simulink model "test_pos_ctrl_target_for_each"  (R2014a)
settings: Solver=ode5  StartTime=0.0  StopTime=inf  FixedStep=basic_time_step  RelTol=1e-3
values from neighbouring files (symbols this model uses):
  basic_time_step = 0.002    [init_pos_ctrl_target_for_each.m]
  g = 9.81    [init_pos_ctrl_target_for_each.m]
  kd = [2 0 0 ... (first row only)    [init_pos_ctrl_target_for_each.m]
  KDP = 11/5    (= 2.2)    [init_pos_ctrl_target_for_each.m]
  KDR = 11/5    (= 2.2)    [init_pos_ctrl_target_for_each.m]
  KDY = 11    [init_pos_ctrl_target_for_each.m]
  ki = 0*[.1 0 0 ... (first row only)    [init_pos_ctrl_target_for_each.m]
  kp = [1 0 0 ... (first row only)    [init_pos_ctrl_target_for_each.m]
  KPP = 30/5    (= 6)    [init_pos_ctrl_target_for_each.m]
  KPR = 30/5    (= 6)    [init_pos_ctrl_target_for_each.m]
  KPY = 30    [init_pos_ctrl_target_for_each.m]
  m0 = 1.3    [init_pos_ctrl_target_for_each.m]
  max_pitch = sin(15*pi/180)    [init_pos_ctrl_target_for_each.m]
  max_roll = sin(15*pi/180)    [init_pos_ctrl_target_for_each.m]
  n_robots = 1    [init_pos_ctrl_target_for_each.m]
undefined symbols (not defined in the file or in its folder): DiscIntNeverNeededParam, IMU_time_step, VICON_time_step
libraries: geometry_msgs x3, sensor_msgs x1, rt_sync x1
settings Model: Creator=prg  LastModifiedBy=fschiano
settings OptimizationCC: ExpressionDepthLimit=2147483647
settings DebuggingCC: UnderspecifiedInitializationDetection=Classic  StateNameClashWarn=warning

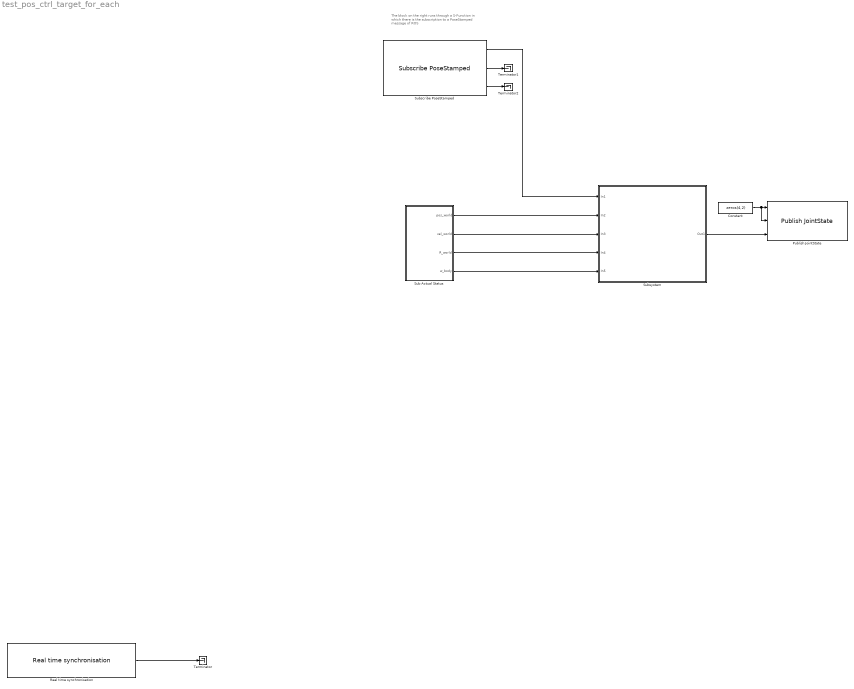
== system test_pos_ctrl_target_for_each ==
  note: The block on the right runs through a S-Function
      | in which there is the subscription to a PoseStamped
      | message of ROS
  Constant : Constant  Value=zeros(4,2)
  Publish JointState : sensor_msgs/Publish JointState  stepTime=basic_time_step  topic_prefix='/command/quadrotor_'  list_of_robot_ids=char([0:1])  topic_postfix=''  n_dofs=char(4)
  Real time synchronisation : rt_sync/Real time synchronisation  stepTime=basic_time_step  minShownDelay=0.5  ShowEveryNumCycles=1/basic_time_step  slowDownFactor=1
  Sub Actual Status : Subsystem
  Subscribe PoseStamped : geometry_msgs/Subscribe PoseStamped  stepTime=basic_time_step  topic_prefix='/vrep/Quadricopter_target_'  list_of_robot_ids=char([0:1])  topic_postfix='/pose'
  Subsystem : Subsystem
  Terminator : Terminator
  Terminator1 : Terminator
  Terminator2 : Terminator
  wires:
  Constant/1 -> Publish JointState/2, Publish JointState/1
  Real time synchronisation/1 -> Terminator/1
  Subscribe PoseStamped/2 -> Terminator1/1
  Subscribe PoseStamped/3 -> Terminator2/1
  Subscribe PoseStamped/1 -> Subsystem/1(In1)
  Sub Actual Status/1(pos_world) -> Subsystem/2(In2)
  Sub Actual Status/2(vel_world) -> Subsystem/3(In3)
  Sub Actual Status/3("R_world ") -> Subsystem/4(In4)
  Sub Actual Status/4(w_body) -> Subsystem/5(In5)
  Subsystem/1(Out1) -> Publish JointState/3

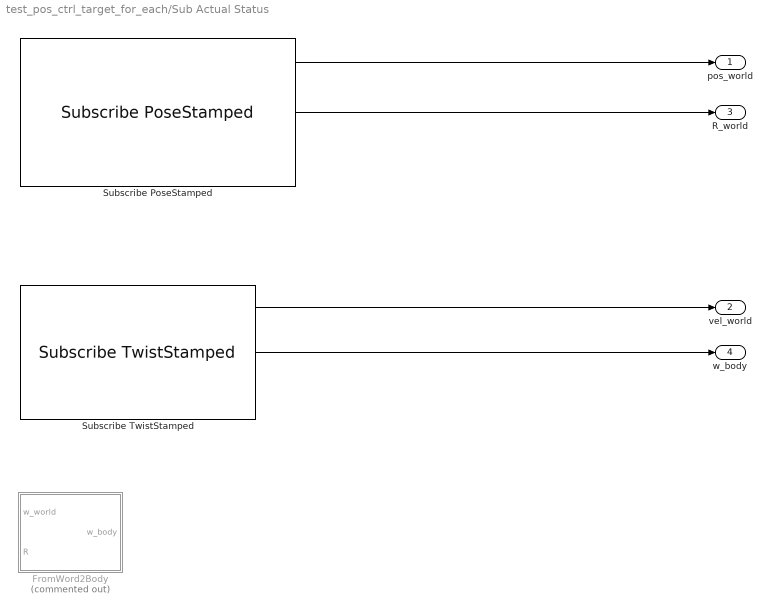
== system test_pos_ctrl_target_for_each/Sub Actual Status ==
  FromWord2Body : MATLAB Function  Commented=on  TreatAsAtomicUnit=on
  Subscribe PoseStamped : geometry_msgs/Subscribe PoseStamped  stepTime=basic_time_step  topic_prefix='/vrep/pose/quadrotor_'  list_of_robot_ids=char([0:1])  topic_postfix=''
  Subscribe TwistStamped : geometry_msgs/Subscribe TwistStamped  stepTime=basic_time_step  topic_prefix='/vrep/twist/quadrotor_'  list_of_robot_ids=char([0:1])  topic_postfix=''
  pos_world : Outport
  vel_world : Outport  Port=2
  "R_world " : Outport  Port=3
  w_body : Outport  Port=4
  wires:
  Subscribe PoseStamped/1 -> pos_world/1
  Subscribe PoseStamped/2 -> "R_world "/1
  Subscribe TwistStamped/1 -> vel_world/1
  Subscribe TwistStamped/2 -> w_body/1

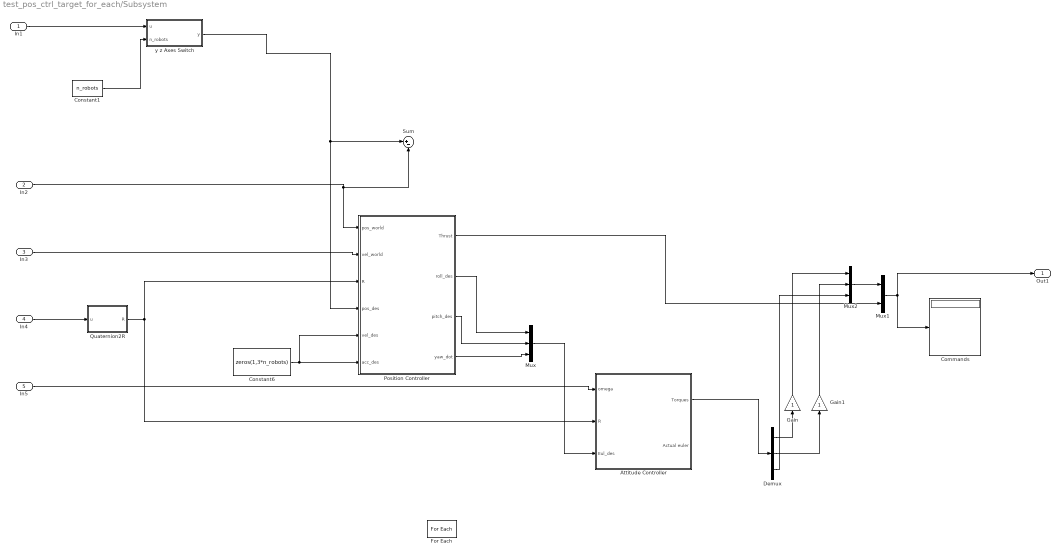
== system test_pos_ctrl_target_for_each/Subsystem ==
  In1 : Inport  Partition=on  PartitionDimension=2  PartitionWidth=1
  In2 : Inport  Port=2  Partition=on  PartitionDimension=2  PartitionWidth=1
  In3 : Inport  Port=3  Partition=on  PartitionDimension=2  PartitionWidth=1
  In4 : Inport  Port=4  Partition=on  PartitionDimension=2  PartitionWidth=1
  In5 : Inport  Port=5  Partition=on  PartitionDimension=2  PartitionWidth=1
  Attitude Controller : Subsystem  SystemSampleTime=IMU_time_step
  Commands : Display
  Constant1 : Constant  Value=n_robots
  Constant6 : Constant  Value=zeros(1,3*n_robots)
  Demux : Demux  Outputs=3
  For Each : ForEach  DisableCoverage=on  IndexMode=One-based
  Gain : Gain
  Gain1 : Gain
  Mux : Mux  Inputs=3
  Mux1 : Mux  Inputs=2
  Mux2 : Mux  Inputs=3
  Position Controller : Subsystem  SystemSampleTime=VICON_time_step
  Quaternion2R : MATLAB Function  TreatAsAtomicUnit=on
  Sum : Sum  Inputs=|+-
  y z Axes Switch : MATLAB Function  TreatAsAtomicUnit=on
  Out1 : Outport  ConcatenationDimension=2
  wires:
  Demux/2 -> Gain1/1
  Demux/3 -> Mux2/3
  Mux2/1 -> Mux1/1
  Mux1/1 -> Out1/1, Commands/1
  y z Axes Switch/1(y) -> Position Controller/4(pos_des), Sum/1
  Gain1/1 -> Mux2/2
  In3/1 -> Position Controller/2(vel_world)
  In4/1 -> Quaternion2R/1(u)
  Position Controller/1(Thrust) -> Mux1/2
  In2/1 -> Sum/2, Position Controller/1(pos_world)
  Position Controller/4(yaw_dot) -> Mux/3
  Constant6/1 -> Position Controller/5(vel_des), Position Controller/6(acc_des)
  Mux/1 -> Attitude Controller/3(Eul_des)
  Demux/1 -> Gain/1
  Position Controller/2(roll_des) -> Mux/1
  Position Controller/3(pitch_des) -> Mux/2
  Gain/1 -> Mux2/1
  Constant1/1 -> y z Axes Switch/2(n_robots)
  Attitude Controller/1(Torques) -> Demux/1
  In5/1 -> Attitude Controller/1(omega)
  In1/1 -> y z Axes Switch/1(u)
  Quaternion2R/1(R) -> Attitude Controller/2(R), Position Controller/3(R)

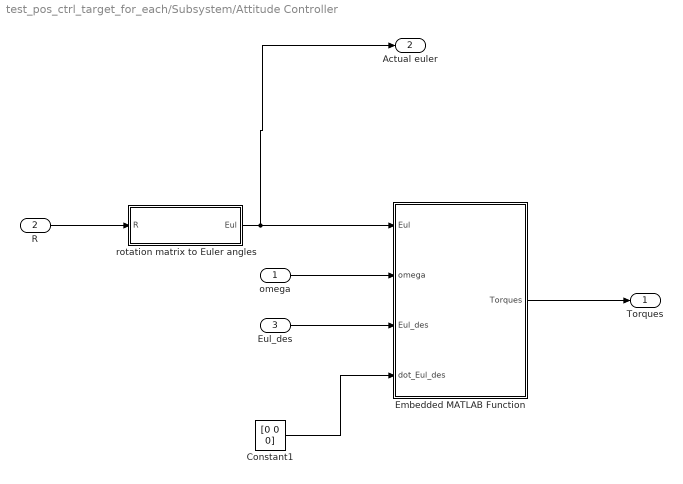
== system test_pos_ctrl_target_for_each/Subsystem/Attitude Controller ==
  omega : Inport
  R : Inport  Port=2
  Eul_des : Inport  Port=3
  Constant1 : Constant  Value=[0 0 0]
  Embedded MATLAB Function : MATLAB Function  TreatAsAtomicUnit=on
  rotation matrix to Euler angles : MATLAB Function  TreatAsAtomicUnit=on
  Torques : Outport
  Actual euler : Outport  Port=2
  wires:
  R/1 -> rotation matrix to Euler angles/1(R)
  rotation matrix to Euler angles/1(Eul) -> Embedded MATLAB Function/1(Eul), Actual euler/1
  omega/1 -> Embedded MATLAB Function/2(omega)
  Eul_des/1 -> Embedded MATLAB Function/3(Eul_des)
  Embedded MATLAB Function/1(Torques) -> Torques/1
  Constant1/1 -> Embedded MATLAB Function/4(dot_Eul_des)

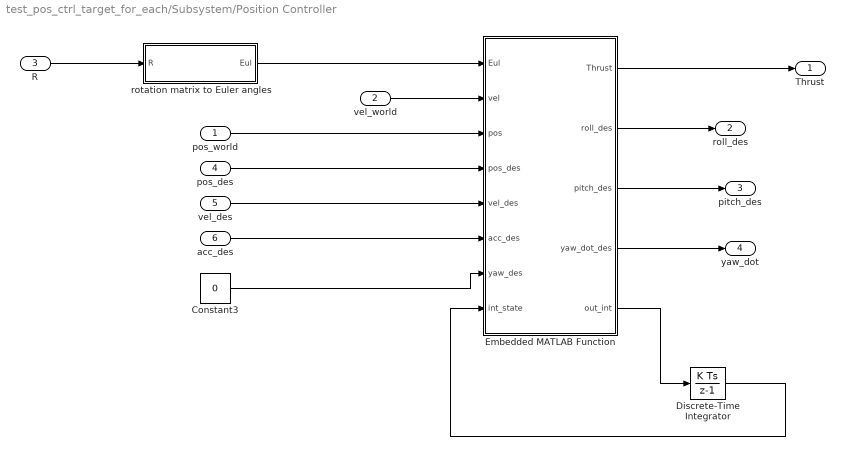
== system test_pos_ctrl_target_for_each/Subsystem/Position Controller ==
  pos_world : Inport
  vel_world : Inport  Port=2
  R : Inport  Port=3
  pos_des : Inport  Port=4
  vel_des : Inport  Port=5
  acc_des : Inport  Port=6
  Constant3 : Constant  Value=0
  Discrete-Time Integrator : DiscreteIntegrator  InitialCondition=[0 0 0]  SampleTime=-1  ICPrevOutput=DiscIntNeverNeededParam  ICPrevScaledInput=DiscIntNeverNeededParam
  Embedded MATLAB Function : MATLAB Function  TreatAsAtomicUnit=on
  rotation matrix to Euler angles : MATLAB Function  TreatAsAtomicUnit=on
  Thrust : Outport
  roll_des : Outport  Port=2
  pitch_des : Outport  Port=3
  yaw_dot : Outport  Port=4
  wires:
  R/1 -> rotation matrix to Euler angles/1(R)
  rotation matrix to Euler angles/1(Eul) -> Embedded MATLAB Function/1(Eul)
  vel_world/1 -> Embedded MATLAB Function/2(vel)
  pos_world/1 -> Embedded MATLAB Function/3(pos)
  Embedded MATLAB Function/1(Thrust) -> Thrust/1
  pos_des/1 -> Embedded MATLAB Function/4(pos_des)
  vel_des/1 -> Embedded MATLAB Function/5(vel_des)
  acc_des/1 -> Embedded MATLAB Function/6(acc_des)
  Constant3/1 -> Embedded MATLAB Function/7(yaw_des)
  Embedded MATLAB Function/2(roll_des) -> roll_des/1
  Embedded MATLAB Function/3(pitch_des) -> pitch_des/1
  Embedded MATLAB Function/4(yaw_dot_des) -> yaw_dot/1
  Embedded MATLAB Function/5(out_int) -> Discrete-Time Integrator/1
  Discrete-Time Integrator/1 -> Embedded MATLAB Function/8(int_state)

== matlab function test_pos_ctrl_target_for_each/Subsystem/Attitude Controller/Embedded MATLAB Function ==
  data: Eul input; Torques output; omega input; Eul_des input; dot_Eul_des input; KDR parameter; KPR parameter; KDP parameter; KPP parameter; KDY parameter; KPY parameter
function Torques  = fcn(Eul, omega, Eul_des, dot_Eul_des, KDR, KPR, KDP, KPP, KDY, KPY)
% This block supports the Embedded MATLAB subset.
% See the help menu for details. 

% p = angles(2);
% r = angles(1);
% y=angles(3);
% 
% T = [1      tan(p)*sin(r) tan(p)*cos(r);
%     0       cos(r)  -sin(r);
%     0       sin(r)/cos(p)   cos(r)/cos(p)];
% 
% dot_ang = T*omega;
% dot_r=dot_ang(1);
% dot_p = dot_ang(2);
% 
% T_dot = [0  tan(p)*cos(r)*dot_r+(sin(r)+tan(p)^2*sin(r))*dot_p -tan(p)*sin(r)*dot_r+(cos(r)+tan(p)^2*cos(r))*dot_p;
%          0  -sin(r)*dot_r   -cos(r)*dot_r;
%          0  cos(r)/cos(p)*dot_r+sin(r)*sin(p)/cos(p)^2*dot_p    -sin(r)/cos(p)*dot_r+cos(r)*sin(p)/cos(p)^2*dot_p];
% 
% 
% k_d = 11;
% k_p = 30;
% ang_vel_des = [0 0 yaw_dot_des]';
% 
% 
% if(yaw_des - angles(3) > pi)
%     angles(3) = angles(3)+2*pi;
% elseif (yaw_des - angles(3) < -pi)
%     angles(3) = angles(3)-2*pi;
% end
% 
% ang_des = [roll_des pitch_des yaw_des]';
% U = I*inv(T)*(k_d*(ang_vel_des-dot_ang)+k_p*(ang_des - angles)-T_dot*omega)+cross(omega, I*omega);
% r_c = U(1);
% p_c = U(2);
% y_c = U(3);

Torques=[0;0;0];

r = Eul(1);
p = Eul(2);
y = Eul(3);




T = [1      tan(p)*sin(r) tan(p)*cos(r);
    0       cos(r)  -sin(r);
    0       sin(r)/cos(p)   cos(r)/cos(p)];


% T=eye(3);

dot_Eul = T*omega;

dot_r = dot_Eul(1);
dot_p = dot_Eul(2);
dot_y = dot_Eul(3);

% U=I*inv(T)*([ KDR * (0 - dot_r) + KPR * (roll_des - r); KDP * (0 - dot_p) + KPP * (pitch_des - p) ; KPY * (yaw_dot_des - dot_y) ]);


Torques(1) = KDR * (dot_Eul_des(1) - dot_r) + KPR * (Eul_des(1) - r);
Torques(2) = KDP * (dot_Eul_des(2) - dot_p) + KPP * (Eul_des(2) - p);
Torques(3) = KDY * (dot_Eul_des(3) - dot_y) + KPY * (Eul_des(3) - y);


% if abs(Torques(1)) > 0.02
%     Torques(1)= 0.02;
%     
% end
% 
% 
% if abs(Torques(2)) > 0.02
%     Torques(2)= 0.02;
%     
% end

== matlab function test_pos_ctrl_target_for_each/Subsystem/Quaternion2R ==
  data: u input; R output
function R = fcn(u)


   



w = u( 1 );
x = u( 2 );
y = u( 3 );
z = u( 4 );

n = sqrt(x*x + y*y + z*z + w*w);


    x = x/ n;
    y = y/ n;
    z = z/ n;
    w = w/ n;

Rxx = 1 - 2*(y^2 + z^2);
Rxy = 2*(x*y - z*w);
Rxz = 2*(x*z + y*w);

Ryx = 2*(x*y + z*w);
Ryy = 1 - 2*(x^2 + z^2);
Ryz = 2*(y*z - x*w );

Rzx = 2*(x*z - y*w );
Rzy = 2*(y*z + x*w );
Rzz = 1 - 2 *(x^2 + y^2);

R = [ 
    Rxx,    Rxy,    Rxz;
    Ryx,    Ryy,    Ryz;
    Rzx,    Rzy,    Rzz];

% 
% 
% a = u( 1 );
% b = u( 2 );
% c = u( 3 );
% d = u( 4 );
% 
% 
%   R(1,1) = a*a+b*b-c*c-d*d;
%   R(1,2) = 2*b*c-2*a*d;
%   R(1,3) = 2*a*c+2*b*d;
%   
%   R(2,1)   = 2*a*d+2*b*c;
%   R(2,2)  = a*a-b*b+c*c-d*d;
%   R(2,3)  = 2*c*d-2*a*b;
%    
%   R(3,1)    = 2*b*d-2*a*c;
%   R(3,2)    = 2*a*b+2*c*d;
%   R(3,3)    = a*a-b*b-c*c+d*d;
% 
%

== matlab function test_pos_ctrl_target_for_each/Subsystem/Position Controller/Embedded MATLAB Function ==
  data: Eul input; Thrust output; roll_des output; pitch_des output; yaw_dot_des output; vel input; pos input; pos_des input; vel_des input; acc_des input; yaw_des input; int_state input; m0 parameter; g parameter; out_int output; kd parameter; kp parameter; ki parameter; max_roll parameter; max_pitch parameter
function [Thrust, roll_des, pitch_des, yaw_dot_des, out_int]  = fcn(Eul, vel, pos, pos_des, vel_des, acc_des, yaw_des, int_state, m0, g, kd, kp, ki, max_roll, max_pitch)
% This block supports the Embedded MATLAB subset
% See the help menu for details. 


r = Eul(1);
p = Eul(2);
y = Eul(3);



Thrust=m0/(cos(r)*cos(p))*(-g + acc_des(3) + kd(3,3)*(vel_des(3) -vel(3)) + kp(3,3)*(pos_des(3)-pos(3)) + int_state(3) );


out_int=ki*(pos_des-pos);



% max_T=30;
% 
% if abs(T(3))>max_T
%     T(3)=sign(T(3))*max_T;
% end

if (Thrust>-5)
    Thrust=-5;
end


if (Thrust<-2*m0*g+5)
    Thrust=-2*m0*g+5;
end




% roll_des=-m/T(3)*( acc_des(2) + kd*(vel_des(2) -vel(2)) + kp*(pos_des(2)-pos(2)) );
% pitch_des=m/T(3)*( acc_des(1) + kd*(vel_des(1) -vel(1)) + kp*(pos_des(1)-pos(1)) );


ddpx=kd(1,1)*(vel_des(1) -vel(1)) + kp(1,1)*(pos_des(1)-pos(1) + int_state(1) );
ddpy=kd(2,2)*(vel_des(2) -vel(2)) + kp(2,2)*(pos_des(2)-pos(2) + int_state(2) );



ctrl_roll=m0/Thrust*( -sin(y)*ddpx+cos(y)*ddpy);

if abs(ctrl_roll)>max_roll
    ctrl_roll=sign(ctrl_roll)*max_roll;
end

ctrl_pitch= m0/(Thrust*cos(r))*( cos(y)*ddpx+sin(y)*ddpy);


if abs(ctrl_pitch)>max_pitch
    ctrl_pitch=sign(ctrl_pitch)*max_pitch;
end





roll_des = -asin( ctrl_roll );

pitch_des = asin(  ctrl_pitch );

yaw_dot_des = 0; % kp(3,3)*(yaw_des-y);

== matlab function test_pos_ctrl_target_for_each/Subsystem/Position Controller/rotation matrix to Euler angles ==
  data: R input; Eul output
function Eul = eulerangles(R)
% This block supports an embeddable subset of the MATLAB language.
% See the help menu for details. 

Roll = atan2(R(3,2),R(3,3));
Pitch = atan2(-R(3,1),sqrt(R(3,2)^2+R(3,3)^2));
Yaw = atan2(R(2,1),R(1,1));


Eul = [Roll; Pitch; Yaw];

== matlab function test_pos_ctrl_target_for_each/Sub Actual Status/FromWord2Body ==
  data: w_world input; w_body output; R input
function w_body = fcn(w_world,R)




w_body = R * w_world;

== matlab function test_pos_ctrl_target_for_each/Subsystem/y z Axes Switch ==
  data: u input; y output; n_robots input
function y = fcn(u,n_robots)
%#codegen

% Transform a matrix (N x N) into a vector ((N*N) X 1)
% To understand how it works try the following lines in MATLAB
% A_example=[1 2 3;4 5 6;7 8 9;10 11 12]
% A_example_vectorized=(A_example(:))

u_vectorized=u(:);
y=u_vectorized;

for i=0:n_robots-1
    for j=2:3
        y((j)+3*i)=-u_vectorized((j)+3*i);
    end
end

== matlab function test_pos_ctrl_target_for_each/Subsystem/Attitude Controller/rotation matrix to Euler angles ==
  data: R input; Eul output
function Eul = eulerangles(R)
% This block supports an embeddable subset of the MATLAB language.
% See the help menu for details. 

Roll = atan2(R(3,2),R(3,3));
Pitch = atan2(-R(3,1),sqrt(R(3,2)^2+R(3,3)^2));
Yaw = atan2(R(2,1),R(1,1));


Eul = [Roll; Pitch; Yaw];
